simulink library "RollRefAssess_Req1_3"  (R2015b)
settings: Solver=VariableStepAuto  StartTime=0.0  StopTime=10.0  RelTol=1e-3
libraries: simulink x8, sldvlib x4
settings Model: Creator=The MathWorks, Inc.  LastModifiedBy=The MathWorks, Inc.
settings HardwareCC: ProdWordSize=32

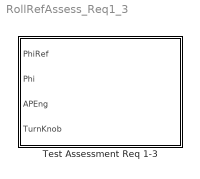
== system RollRefAssess_Req1_3 ==
  Test Assessment Req 1-3 : Subsystem

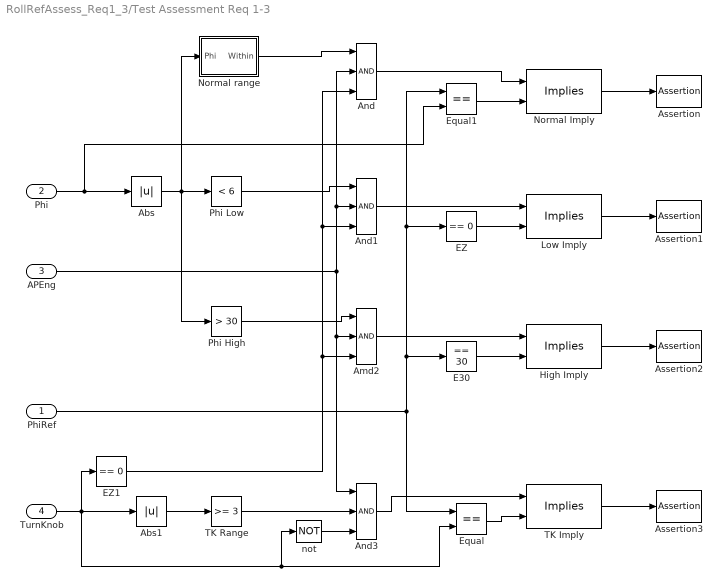
== system RollRefAssess_Req1_3/Test Assessment Req 1-3 ==
  PhiRef : Inport
  Phi : Inport  Port=2
  APEng : Inport  Port=3
  TurnKnob : Inport  Port=4
  Abs : Abs
  Abs1 : Abs
  Amd2 : Logic  Inputs=3  AllPortsSameDT=off  OutDataTypeStr=boolean
  And : Logic  Inputs=3  AllPortsSameDT=off  OutDataTypeStr=boolean
  And1 : Logic  Inputs=3  AllPortsSameDT=off  OutDataTypeStr=boolean
  And3 : Logic  Inputs=3  AllPortsSameDT=off  OutDataTypeStr=boolean
  Assertion : Assertion  AssertionFailFcn=disp(sprintf('\nPhiRef must = Phi when Phi in normal range.'))  StopWhenAssertionFail=off
  Assertion1 : Assertion  AssertionFailFcn=disp(sprintf('\nPhiRef must = 0 when Phi < 6 deg.'))  StopWhenAssertionFail=off
  Assertion2 : Assertion  AssertionFailFcn=disp(sprintf('\nFailure of high limit test.\nPhiRef must = 0 when Phi > 30 deg.'))  StopWhenAssertionFail=off
  Assertion3 : Assertion  AssertionFailFcn=disp(sprintf('\nPhiRef must = TK value when TK > 3 deg.'))  StopWhenAssertionFail=off
  E30 : simulink/Logic and Bit Operations/Compare To Constant  relop===  const=30  OutDataTypeStr=boolean
  EZ : simulink/Logic and Bit Operations/Compare To Zero  relop===  OutDataTypeStr=boolean
  EZ1 : simulink/Logic and Bit Operations/Compare To Zero  relop===  OutDataTypeStr=boolean
  Equal : RelationalOperator  Operator===  OutDataTypeStr=boolean
  Equal1 : RelationalOperator  Operator===  OutDataTypeStr=boolean
  High Imply : sldvlib/Verification Utilities/Implies
  Low Imply : sldvlib/Verification Utilities/Implies
  Normal Imply : sldvlib/Verification Utilities/Implies
  Normal range : Subsystem
  Phi High : simulink/Logic and Bit Operations/Compare To Constant  relop=>  const=30  OutDataTypeStr=boolean
  Phi Low : simulink/Logic and Bit Operations/Compare To Constant  relop=<  const=6  OutDataTypeStr=boolean
  TK Imply : sldvlib/Verification Utilities/Implies
  TK Range : simulink/Logic and Bit Operations/Compare To Constant  relop=>=  const=3  OutDataTypeStr=boolean
  not : Logic  Operator=NOT  Inputs=1  AllPortsSameDT=off  OutDataTypeStr=boolean
  wires:
  APEng/1 -> And3/1, Amd2/2, And/2, And1/2
  Phi/1 -> Equal1/2, Abs/1
  Phi Low/1 -> And1/1
  EZ/1 -> Low Imply/2
  PhiRef/1 -> E30/1, Equal1/1, EZ/1, Equal/1
  And1/1 -> Low Imply/1
  Phi High/1 -> Amd2/1
  E30/1 -> High Imply/2
  Amd2/1 -> High Imply/1
  Abs/1 -> Normal range/1(Phi), Phi High/1, Phi Low/1
  Abs1/1 -> TK Range/1
  TK Range/1 -> And3/2
  And3/1 -> TK Imply/1
  Equal/1 -> TK Imply/2
  Normal range/1(Within) -> And/1
  Equal1/1 -> Normal Imply/2
  And/1 -> Normal Imply/1
  Low Imply/1 -> Assertion1/1
  High Imply/1 -> Assertion2/1
  TK Imply/1 -> Assertion3/1
  Normal Imply/1 -> Assertion/1
  EZ1/1 -> Amd2/3, And1/3, And/3
  TurnKnob/1 -> EZ1/1, not/1, Equal/2, Abs1/1
  not/1 -> And3/3

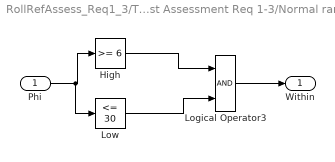
== system RollRefAssess_Req1_3/Test Assessment Req 1-3/Normal range ==
  Phi : Inport
  High : simulink/Logic and Bit Operations/Compare To Constant  relop=>=  const=6  OutDataTypeStr=boolean
  Logical Operator3 : Logic  AllPortsSameDT=off  OutDataTypeStr=boolean
  Low : simulink/Logic and Bit Operations/Compare To Constant  relop=<=  const=30  OutDataTypeStr=boolean
  Within : Outport
  wires:
  Low/1 -> Logical Operator3/2
  Phi/1 -> Low/1, High/1
  High/1 -> Logical Operator3/1
  Logical Operator3/1 -> Within/1
